simulink model "simulate_sensors"  (R2025a)
settings: Solver=FixedStepAuto  StartTime=0.0  StopTime=20  FixedStep=0.0001  RelTol=1e-3
undefined symbols (not defined in the file or in its folder): fractalcoef
libraries: sensorgpslib x1, mspsensorlib x1
settings Model: Creator=jonno  LastModifiedBy=jonno

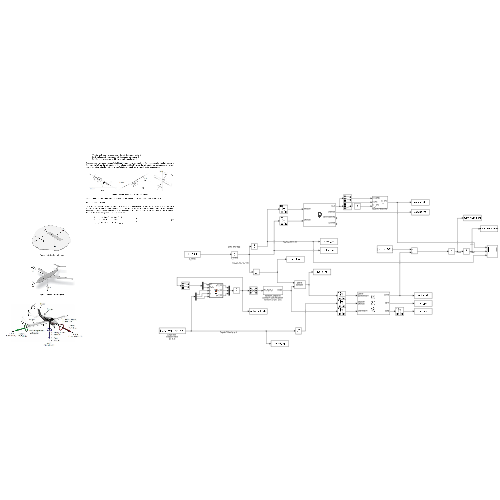
[thumbnail: Simulink's stored preview of the top-level diagram]
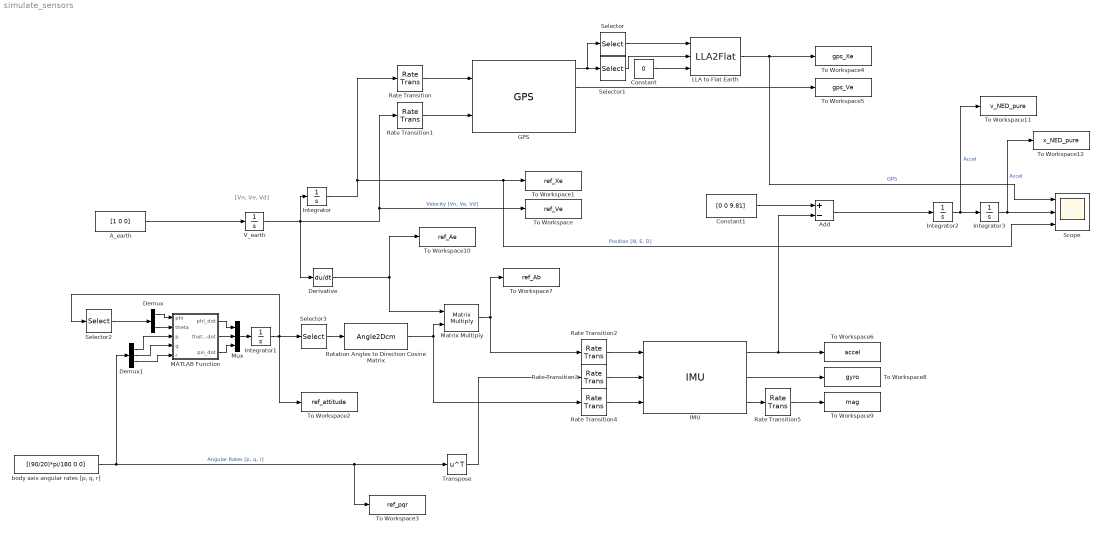
== system simulate_sensors ==
  note: [Vn, Ve, Vd]
  A_earth : Constant  Value=[1 0 0]  VectorParams1D=off
  Add : Sum  Inputs=+-
  Constant : Constant  Value=0
  Constant1 : Constant  Value=[0 0 9.81]
  Demux : Demux  Outputs=2
  Demux1 : Demux  Outputs=3
  Derivative : Derivative
  GPS : sensorgpslib/GPS  DispRefFrame=NED  PositionInputFormat=Local  ReferenceLocation=[ 0, 0, 0 ]  HorizontalPositionAccuracy=1.6  VerticalPositionAccuracy=3  VelocityAccuracy=0.1  DecayFactor=0.999  SeedDouble=67  SimulateUsing=Interpreted execution
      settings: LibrarySourceBlock=mspsensorlib/GPS
  IMU : mspsensorlib/IMU  DispRefFrame=NED  TemperaturePort=off  Temperature=25  MagneticFieldPort=off  MagneticFieldNED=[ 27.5550, -2.4169, -16.0849 ]  MagneticFieldENU=[ -2.4169, 27.5550, 16.0849 ]  SeedDouble=67  SimulateUsing=Code generation  AccelParamsMeasurementRange=16*9.81  AccelParamsResolution=((0.732)/1000)*9.81  AccelParamsConstantBias=[0 0.0 0.0]  AccelParamsAxesMisalignment=[0 0 0]  AccelParamsNoiseDensity=[0.37 0.37 0.37]  AccelParamsBiasInstability=[0 0 0]  AccelParamsBiasInstabilityNumerator=fractalcoef().Numerator  AccelParamsBiasInstabilityDenominator=fractalcoef().Denominator  AccelParamsRandomWalk=[0 0 0]  AccelParamsNoiseType=double-sided  AccelParamsTemperatureBias=[0 0 0]  AccelParamsTemperatureScaleFactor=[0 0 0]  GyroParamsMeasurementRange=34.9066  GyroParamsResolution=0.0017453  GyroParamsConstantBias=[0 0 0]  GyroParamsAxesMisalignment=0  GyroParamsAccelerationBias=[2.72e-05 2.72e-05 2.72e-05]  GyroParamsNoiseDensity=[9.89e-05 9.89e-05 9.89e-05]  GyroParamsBiasInstability=[3.88e-04 3.88e-04 3.88e-04]  GyroParamsBiasInstabilityNumerator=fractalcoef().Numerator  GyroParamsBiasInstabilityDenominator=fractalcoef().Denominator  GyroParamsRandomWalk=[0 0 0]  GyroParamsNoiseType=double-sided  GyroParamsTemperatureBias=[0 0 0]  GyroParamsTemperatureScaleFactor=[0 0 0]  MagParamsMeasurementRange=800  MagParamsResolution=0.025  MagParamsConstantBias=0  MagParamsAxesMisalignment=[0 0 0]  MagParamsNoiseDensity=[0.06 0.06 0.06]  MagParamsBiasInstability=[0 0 0]  MagParamsBiasInstabilityNumerator=fractalcoef().Numerator  MagParamsBiasInstabilityDenominator=fractalcoef().Denominator  MagParamsRandomWalk=[0 0 0]  MagParamsNoiseType=double-sided  MagParamsTemperatureBias=[0 0 0]  MagParamsTemperatureScaleFactor=[0 0 0]
  Integrator : Integrator  InitialCondition=[0, 0, 0]
  Integrator1 : Integrator  InitialCondition=[0 0 0]
  Integrator2 : Integrator
  Integrator3 : Integrator
  LLA to Flat Earth : LLA2Flat  LL0=[0 0]
  MATLAB Function : MATLAB Function  TreatAsAtomicUnit=on
  Matrix Multiply : Product  Multiplication=Matrix(*)
  Mux : Mux  Inputs=3
  Rate Transition : RateTransition  OutPortSampleTime=1/20
  Rate Transition1 : RateTransition  OutPortSampleTime=1/20
  Rate Transition2 : RateTransition  OutPortSampleTime=1/400
  Rate Transition3 : RateTransition  OutPortSampleTime=1/400
  Rate Transition4 : RateTransition  OutPortSampleTime=1/400
  Rate Transition5 : RateTransition  OutPortSampleTime=1/200
  Rotation Angles to Direction Cosine Matrix : Angle2Dcm
      settings: AttributesFormatString=Rotation Order: %<rotationOrder>
  Scope : Scope  NumInputPorts=3
      settings: ActiveDisplayYMinimum=-216.43260042470644  ActiveDisplayYMaximum=808.90474798733931
  Selector : Selector  InputPortWidth=3  IndexOptions=Index vector (dialog)  Indices=[1 2]  OutputSizes=1
  Selector1 : Selector  InputPortWidth=3  IndexOptions=Index vector (dialog)  Indices=[3]  OutputSizes=1
  Selector2 : Selector  InputPortWidth=3  IndexOptions=Index vector (dialog)  Indices=[1 2]  OutputSizes=1
  Selector3 : Selector  InputPortWidth=3  IndexOptions=Index vector (dialog)  Indices=[3 2 1]  OutputSizes=1
  To Workspace : ToWorkspace  VariableName=ref_Ve  SaveFormat=Timeseries  SampleTime=-1
  To Workspace1 : ToWorkspace  VariableName=ref_Xe  SaveFormat=Timeseries  SampleTime=-1
  To Workspace10 : ToWorkspace  VariableName=ref_Ae  SaveFormat=Timeseries  SampleTime=-1
  To Workspace11 : ToWorkspace  VariableName=v_NED_pure  SaveFormat=Timeseries  SampleTime=-1
  To Workspace12 : ToWorkspace  VariableName=x_NED_pure  SaveFormat=Timeseries  SampleTime=-1
  To Workspace2 : ToWorkspace  VariableName=ref_attitude  SaveFormat=Timeseries  SampleTime=-1
  To Workspace3 : ToWorkspace  VariableName=ref_pqr  SaveFormat=Timeseries  SampleTime=-1
  To Workspace4 : ToWorkspace  VariableName=gps_Xe  SaveFormat=Timeseries  SampleTime=-1
  To Workspace5 : ToWorkspace  VariableName=gps_Ve  SaveFormat=Timeseries  SampleTime=-1
  To Workspace6 : ToWorkspace  VariableName=accel  SaveFormat=Timeseries  SampleTime=-1
  To Workspace7 : ToWorkspace  VariableName=ref_Ab  SaveFormat=Timeseries  SampleTime=-1
  To Workspace8 : ToWorkspace  VariableName=gyro  SaveFormat=Timeseries  SampleTime=-1
  To Workspace9 : ToWorkspace  VariableName=mag  SaveFormat=Timeseries  SampleTime=-1
  Transpose : Math  Operator=transpose
  V_earth : Integrator
  "body axis angular rates [p, q, r]" : Constant  Value=[(90/20)*pi/180 0 0]
  wires:
  V_earth/1 -> Derivative/1, To Workspace/1, Rate Transition1/1, Integrator/1  "Velocity [Vn, Ve, Vd]"
  Integrator/1 -> Scope/3, To Workspace1/1, Rate Transition/1  "Position [N, E, D]"
  "body axis angular rates [p, q, r]"/1 -> Transpose/1, To Workspace3/1, Demux1/1  "Angular Rates [p, q, r]"
  Rate Transition/1 -> GPS/1
  Rate Transition1/1 -> GPS/2
  GPS/1 -> Selector/1, Selector1/1
  Selector/1 -> LLA to Flat Earth/1
  Selector1/1 -> LLA to Flat Earth/2
  Constant/1 -> LLA to Flat Earth/3
  GPS/2 -> To Workspace5/1
  Matrix Multiply/1 -> To Workspace7/1, Rate Transition2/1
  A_earth/1 -> V_earth/1
  Transpose/1 -> Rate Transition3/1
  Derivative/1 -> To Workspace10/1, Matrix Multiply/1
  Rate Transition2/1 -> IMU/1
  Rate Transition3/1 -> IMU/2
  IMU/2 -> To Workspace8/1
  IMU/1 -> Add/2, To Workspace6/1
  Rate Transition4/1 -> IMU/3
  Rotation Angles to Direction Cosine Matrix/1 -> Rate Transition4/1, Matrix Multiply/2
  MATLAB Function/1(phi_dot) -> Mux/1
  MATLAB Function/2(theta_dot) -> Mux/2
  MATLAB Function/3(psi_dot) -> Mux/3
  Mux/1 -> Integrator1/1
  Integrator1/1 -> To Workspace2/1, Selector2/1, Selector3/1
  Selector2/1 -> Demux/1
  Demux/2 -> MATLAB Function/2(theta)
  Demux/1 -> MATLAB Function/1(phi)
  Demux1/1 -> MATLAB Function/3(p)
  Demux1/2 -> MATLAB Function/4(q)
  Demux1/3 -> MATLAB Function/5(r)
  Selector3/1 -> Rotation Angles to Direction Cosine Matrix/1
  IMU/3 -> Rate Transition5/1
  Rate Transition5/1 -> To Workspace9/1
  LLA to Flat Earth/1 -> Scope/1, To Workspace4/1  "GPS"
  Add/1 -> Integrator2/1
  Integrator2/1 -> To Workspace11/1, Integrator3/1  "Accel"
  Constant1/1 -> Add/1
  Integrator3/1 -> Scope/2, To Workspace12/1  "Accel"

== matlab function simulate_sensors/MATLAB Function ==
  data: phi input; phi_dot output; theta input; p input; q input; r input; theta_dot output; psi_dot output
function [phi_dot, theta_dot, psi_dot] = fcn(phi, theta, p, q, r)
% Correct transformation matrix from Equation 3.7
transform_matrix = [1   sin(phi)*tan(theta)   cos(phi)*tan(theta);
                    0   cos(phi)              -sin(phi); %<- Corrected this term
                    0   sin(phi)/cos(theta)   cos(phi)/cos(theta)];

% Input vector of body rates
body_rates = [p; q; r];

% Use matrix multiplication (*) instead of element-wise (.*)
euler_rates = transform_matrix * body_rates;

phi_dot   = euler_rates(1);
theta_dot = euler_rates(2);
psi_dot   = euler_rates(3); % Renamed from omega_dot for clarity
